simulink model "step2d"  (Simulink 8.5)
settings: Solver=ode45  SolverMode=SingleTasking  StartTime=0.0  StopTime=3  MaxStep=1e-4  RelTol=1e-4  AbsTol=1e-6
undefined symbols (not defined in the file or in its folder): den, dx, num
libraries: simulink x1
settings Model: Creator=PC  LastModifiedBy=PC
settings DataIOCC: LimitDataPoints=off
settings OptimizationCC: BlockReduction=off  BooleanDataType=off  ExpressionDepthLimit=128
settings DebuggingCC: SaveWithParameterizedLinksMsg=none  SignalResolutionControl=TryResolveAllWithWarning  MultiTaskDSMMsg=warning  MultiTaskCondExecSysMsg=none  FcnCallInpInsideContextMsg=EnableAllAsError  StateNameClashWarn=none  StrictBusMsg=None
settings HardwareCC: TargetUnknown=on
settings RTWCC: TemplateMakefile=grt_vc.tmf

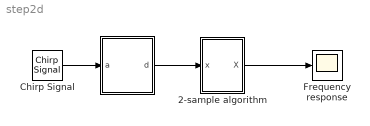
== system step2d ==
  "  " : Subsystem  mask(Data Adquisition Board){filter=on, approx=Butterworth, order=3, numerator=[], denominator=[], freq=180, resdis=on, vertres=8, xmax=100, winsize=2, G=1.0, fs=60*20}
      mask prompts: filter "Disable Analog Filter"; approx "Filter approximation"; numerator "Free expression filter: numerator(descending order of s)"; denominator "Free expression filter: denominator:"; freq "Cut-off frequency"; resdis "Disable Vertical Resolution"; vertres "Vertical Resolution: No. of bits"; xmax "Vertical Resolution: signal range"; winsize "Window size"; G "Gain"; fs "Sampling frequency"
      mask help: Takes the instantaneous value of the input signal and convert it to the data window of samples.
      mask init:
      | dab1
      mask TypeOptions approx: Bessel | Tschebyscheff | Butterworth | free expression
      mask TypeOptions order: 2 | 3 | 4
      mask TypeOptions vertres: 8 | 12 | 16
      mask Display: disp('DAB')
  2-sample algorithm : Subsystem
  Chirp Signal : simulink/Sources/Chirp Signal  f1=0  T=3  f2=180
  Frequency response : Scope
      settings: TickLabels=on  YMin=0  YMax=1.5
  wires:
  "  "/1(d) -> 2-sample algorithm/1(x)
  Chirp Signal/1 -> "  "/1(a)
  2-sample algorithm/1(X) -> Frequency response/1

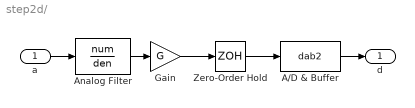
== system step2d/   ==
  a : Inport
  A/D & Buffer : S-Function  FunctionName=dab2  Parameters=winsize,fs,dx,resdis
  Analog Filter : TransferFcn  Numerator=num  Denominator=den
  Gain : Gain  Gain=G  SaturateOnIntegerOverflow=on  OutDataTypeStr=Inherit: Same as input  ParamDataTypeStr=Inherit: Same as input
  Zero-Order Hold : ZeroOrderHold  SampleTime=1/fs
  d : Outport  InitialOutput=[zeros(winsize,1)]
  wires:
  A/D & Buffer/1 -> d/1
  a/1 -> Analog Filter/1
  Zero-Order Hold/1 -> A/D & Buffer/1
  Gain/1 -> Zero-Order Hold/1
  Analog Filter/1 -> Gain/1

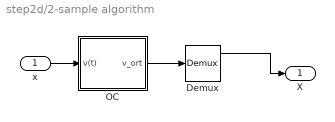
== system step2d/2-sample algorithm ==
  x : Inport
  Demux : Demux  Outputs=2
  OC : Subsystem  mask{tfilt=User Defined, rfilt=[ 1 1]*0.51253, ifilt=[ -1,1]*3.23606, tlen=full, N1=2}
      mask prompts: tfilt "type of filter:"; rfilt "direct filter"; ifilt "quadrature filter"; tlen "type of data window"; N1 "number of samples per cycle:"
      mask help:
      | Input:
      |    input window of the sampled signal (vector with length N1)
      | Output:
      |    orthogonal components (complex)
      | note: the type of data window only affects the Fourier filter only.
      mask Help:
      | This block take the date as its input window of the sampled signal, and convert it into a single orthogonal output. The output values are direct and quadrature orthogonal components of signal at the present sampling instant.
      | The options of the block include type and data window length of pre-defined filters and user-defined filters.
      mask TypeOptions tfilt: Fourier | Walsh | User Defined
      mask TypeOptions tlen: half | full
  X : Outport  InitialOutput=0
  wires:
  x/1 -> OC/1(v(t))
  OC/1(v_ort) -> Demux/1
  Demux/1 -> X/1

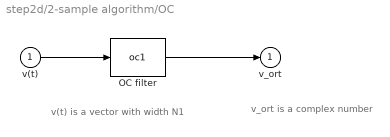
== system step2d/2-sample algorithm/OC ==
  note: v_ort is
      | a complex number
  note: v(t) is a vector
      | with width N1
  v(t) : Inport
  OC filter : S-Function  FunctionName=oc1  Parameters=tfilt, rfilt, ifilt, tlen, N1
  v_ort : Outport  InitialOutput=0
  wires:
  OC filter/1 -> v_ort/1
  v(t)/1 -> OC filter/1
